simulink model "mass_spring_damper"  (R2024b)
settings: Solver=VariableStepAuto  StartTime=0.0  StopTime=5  RelTol=1e-3
undefined symbols (not defined in the file): damping_ratio, natural_frequency
settings Model: Creator=Utilizador  LastModifiedBy=Utilizador

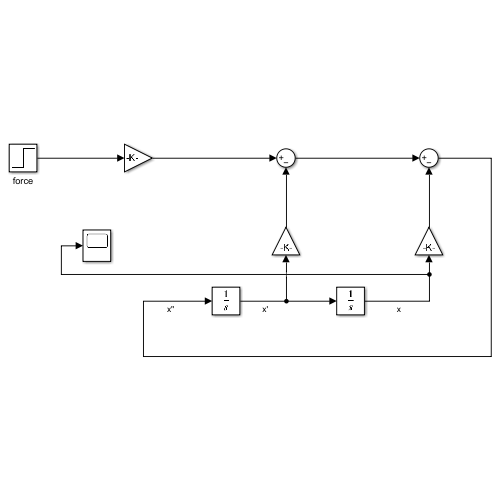
[thumbnail: Simulink's stored preview of the top-level diagram]
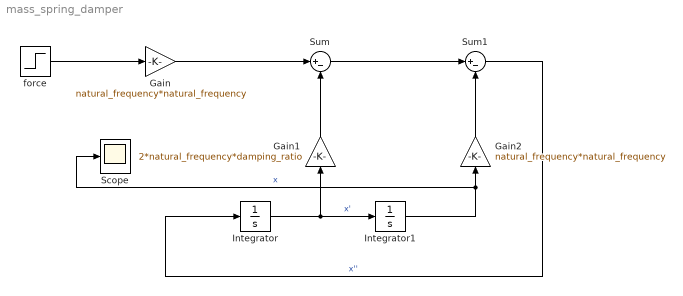
== system mass_spring_damper ==
  Gain : Gain  Gain=natural_frequency*natural_frequency
  Gain1 : Gain  Gain=2*natural_frequency*damping_ratio
  Gain2 : Gain  Gain=natural_frequency*natural_frequency
  Integrator : Integrator
  Integrator1 : Integrator
  Scope : Scope
  Sum : Sum  Inputs=|+-
  Sum1 : Sum  Inputs=|+-
  force : Step  SampleTime=0
  wires:
  Integrator/1 -> Gain1/1, Integrator1/1  "x'"
  Sum1/1 -> Integrator/1  "x''"
  Integrator1/1 -> Gain2/1, Scope/1  "x"
  force/1 -> Gain/1
  Gain/1 -> Sum/1
  Gain1/1 -> Sum/2
  Sum/1 -> Sum1/1
  Gain2/1 -> Sum1/2
